simulink model "Simulink_Observation_5"  (R2020b)
settings: Solver=FixedStepDiscrete  StartTime=0.0  StopTime=0  RelTol=1e-3
settings Model: Creator=Mohit Akhouri  LastModifiedBy=Mohit Akhouri
settings SolverCC: AutoInsertRateTranBlk=on

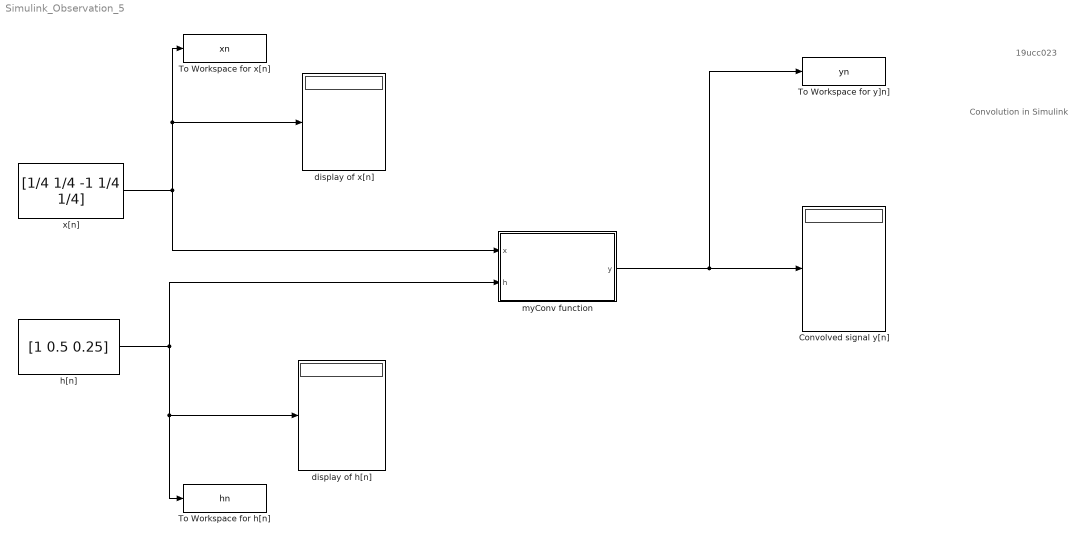
== system Simulink_Observation_5 ==
  note: Convolution in Simulink
  note: 19ucc023
  Convolved signal y[n] : Display
  To Workspace for h[n] : ToWorkspace  VariableName=hn  SaveFormat=Timeseries  SampleTime=-1
  To Workspace for x[n] : ToWorkspace  VariableName=xn  SaveFormat=Timeseries  SampleTime=-1
  To Workspace for y]n] : ToWorkspace  VariableName=yn  SaveFormat=Timeseries  SampleTime=-1
  display of h[n] : Display
  display of x[n] : Display
  h[n] : Constant  Value=[1 0.5 0.25]
  myConv function : MATLAB Function  TreatAsAtomicUnit=on
  x[n] : Constant  Value=[1/4 1/4 -1 1/4 1/4]
  wires:
  h[n]/1 -> To Workspace for h[n]/1, display of h[n]/1, myConv function/2(h)
  x[n]/1 -> myConv function/1(x), To Workspace for x[n]/1, display of x[n]/1
  myConv function/1(y) -> Convolved signal y[n]/1, To Workspace for y]n]/1

== matlab function Simulink_Observation_5/myConv function ==
  data: x input; y output; h input
function y  = fcn(x,h)

% Generating the convolution matrix and finding convolution of
% two finite length sequences x[n] and h[n]

% Computing the Convolution matrix
rows = length(x);
length_h = length(h);
columns = rows + length_h - 1;
M = zeros(rows,columns);

for i=1:rows
    offset = i; % offset in the matrix from where 'h' needs to be stored
    for j=1:length_h
        M(i,offset) = h(j);
        offset = offset + 1; % offset incremented 
    end
end

% computing convolution from Convolution matrix
y = zeros(1,columns);
sum = 0; % temporary variable to store sum

% ALGORITHM for calculation of convolution of sequences is as follows
for i=1:columns
    sum = 0;
    for j=1:rows
       sum = sum + (M(j,i)*x(j));
    end
    y(i) = sum;
end     
end
